simulink model "Lift_problem8"  (R2020b)
settings: Solver=VariableStepAuto  StartTime=0.0  StopTime=10.0  RelTol=1e-3
settings Model: Creator=Sourav Kumar  LastModifiedBy=Sourav Kumar

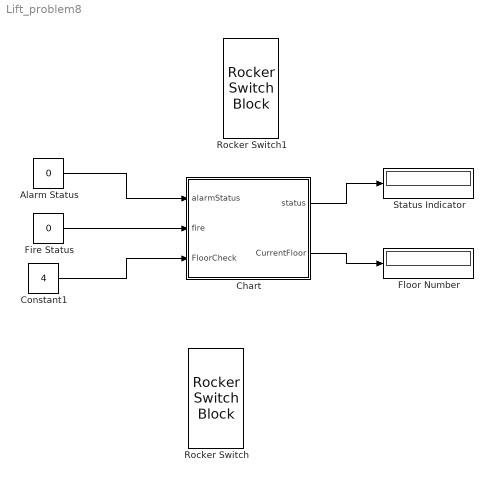
== system Lift_problem8 ==
  Alarm Status : Constant  Value=0
  Chart : Stateflow chart  TreatAsAtomicUnit=on
  Constant1 : Constant  Value=4
  Fire Status : Constant  Value=0
  Floor Number : Display
  Rocker Switch : RockerSwitchBlock
      settings: Values={{'Off', 'On'}, [0 1]}
  Rocker Switch1 : RockerSwitchBlock
      settings: Values={{'Off', 'On'}, [0 1]}
  Status Indicator : Display
  wires:
  Alarm Status/1 -> Chart/1(alarmStatus)
  Constant1/1 -> Chart/3(FloorCheck)
  Fire Status/1 -> Chart/2(fire)
  Chart/1(status) -> Status Indicator/1
  Chart/2(CurrentFloor) -> Floor Number/1

== stateflow chart Lift_problem8/Chart ==
  state LiftOperation [parallel]
    entry:
    status=0;
    settings: executionOrder=1
    state LiftFunctionOn
      (history)
      state GroundFloor
        entry:
        status=1;
        during:
        CurrentFloor=0;
        FloorCheck(CurrentFloor);
        exit:
        status=0;
      state FirstFloor
        entry:
        status=1;
        during:
        CurrentFloor=1;
        FloorCheck(CurrentFloor);
        exit:
        status=0
      state SecondFloor
        entry:
        status=1;
        during:
        CurrentFloor=2;
        FloorCheck(CurrentFloor);
        exit:
        status=0;
        after(1,sec);
      state ThirdFloor
        entry:
        status=1;
        during:
        CurrentFloor=3;
        FloorCheck(CurrentFloor);
        exit:
        status=0;
        after(1,sec);
      state FourthFloor
        entry:
        status=1
        during:
        CurrentFloor=4;
        FloorCheck(CurrentFloor);
        exit:
        status=0;
      state FifthFloor
        entry:
        status=1;
        during:
        CurrentFloor=5;
        FloorCheck(CurrentFloor);
        exit:
        status=0;
      (default) -> GroundFloor
      GroundFloor -> FirstFloor : up
      FirstFloor -> GroundFloor [order 2] : down
      FirstFloor -> SecondFloor [order 1] : up
      SecondFloor -> FirstFloor [order 2] : down
      SecondFloor -> ThirdFloor [order 1] : up
      ThirdFloor -> SecondFloor [order 2] : down
      ThirdFloor -> FourthFloor [order 1] : up
      FourthFloor -> ThirdFloor [order 2] : down
      FourthFloor -> FifthFloor [order 1] : up
      FifthFloor -> FourthFloor : down
    state LiftFunctionOff
      entry:
      status=0;
    (default) -> LiftFunctionOn
    LiftFunctionOff -> LiftFunctionOn : [fire==0]
    LiftFunctionOn -> LiftFunctionOff : [fire==1]
  state Alarm [parallel]
    settings: executionOrder=2
    (default) -> (junction 37)
    (junction 37) -> (junction 38)
    (junction 38) -> (junction 39) [order 1]
    (junction 39) -> (junction 40) [order 2] : [alarmStatus==1]{send(off);}
    (junction 42) -> (junction 38)
    (junction 38) -> (junction 41) [order 2]
    (junction 39) -> (junction 42) [order 1] : [alarmStatus==0]{send(on);}
    (junction 40) -> (junction 43)
    (junction 43) -> (junction 42)
  data: alarmStatus input; fire input; status output; FloorCheck input; CurrentFloor output
  events: down local RISING_EDGE_EVENT; up local RISING_EDGE_EVENT; off local FUNCTION_CALL_EVENT; on local FUNCTION_CALL_EVENT
